simulink model "simulink_base_problemas_clase1"  (R2021a)
settings: Solver=ode4  StartTime=0.0  StopTime=10000  FixedStep=0.01  RelTol=1e-100
values from neighbouring files (symbols this model uses):
  N_dr_H2N_0 = [0;7.6408;0]    [clase1_problemas.m]
  N_r_H2N_0 = [7000;0;0]    [clase1_problemas.m]
settings Model: SimulationMode=accelerator  Creator=Franklin  LastModifiedBy=Franklin

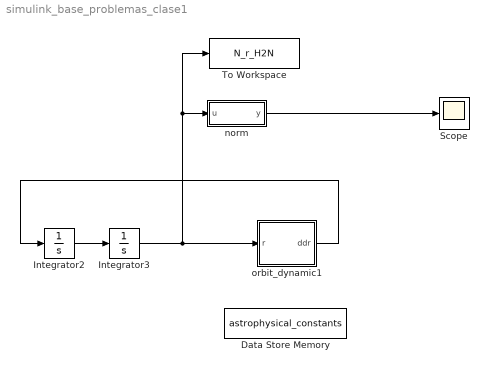
== system simulink_base_problemas_clase1 ==
  Data Store Memory : DataStoreMemory  DataStoreName=astrophysical_constants  ReadBeforeWriteMsg=warning  WriteAfterWriteMsg=warning  WriteAfterReadMsg=warning  InitialValue=astrophysical_constants  ShowAdditionalParam=off  OutDataTypeStr=double
  Integrator2 : Integrator  InitialCondition=N_dr_H2N_0
  Integrator3 : Integrator  InitialCondition=N_r_H2N_0
  Scope : Scope
  To Workspace : ToWorkspace  VariableName=N_r_H2N  SampleTime=10
  norm : MATLAB Function  TreatAsAtomicUnit=on
  orbit_dynamic1 : MATLAB Function  TreatAsAtomicUnit=on
  wires:
  Integrator2/1 -> Integrator3/1
  Integrator3/1 -> To Workspace/1, norm/1(u), orbit_dynamic1/1(r)
  orbit_dynamic1/1(ddr) -> Integrator2/1
  norm/1(y) -> Scope/1

== matlab function simulink_base_problemas_clase1/norm ==
  data: u input; y output
function y = fcn(u)
y = norm(u);

== matlab function simulink_base_problemas_clase1/orbit_dynamic1 ==
  settings: updateMethod=DISCRETE
  data: r input; ddr output; astrophysical_constants data_store_memory
function ddr = fcn(r)
global astrophysical_constants;

mu_earth=astrophysical_constants(1,1);

ddr = -(mu_earth/(norm(r)^3))*r;
